simulink model "kinEq_sim_Explore_Badweh_2nd"  (R2024a)
settings: Solver=FixedStepDiscrete  StartTime=0.0  StopTime=5  FixedStep=TS  RelTol=1e-3  EnableMultiTasking=on
PostLoadFcn:
  | params
model workspace (MAT data in the model file):
  Ia = 0.1
  Id = 0.25
  Pa = 5
  Pd = 9
  TS = 0.01
undefined symbols (not defined in the file): DiscIntNeverNeededParam, L, r, sigbuilder_block, StartTheta, StartX, StartY
libraries: simulink_extras x9
settings Model: Creator=mgovinda  LastModifiedBy=Sheen
settings SolverCC: AlgebraicLoopSolver=TrustRegion
settings DataIOCC: LimitDataPoints=on  SaveFormat=Array  ReturnWorkspaceOutputs=off
settings OptimizationCC: LifeSpan=inf
settings DebuggingCC: UnconnectedInputMsg=warning  UnconnectedOutputMsg=warning  UnconnectedLineMsg=warning  SFUnexpectedBacktrackingDiag=warning  SFNoUnconditionalDefaultTransitionDiag=warning  SFExecutionAtInitializationDiag=none  ArithmeticOperatorsInVariantConditions=warning
settings HardwareCC: ProdBitPerPointer=32  ProdBitPerSizeT=32  ProdBitPerPtrDiffT=32  ProdLargestAtomicFloat=None  ProdIntDivRoundTo=Undefined  ProdEndianess=Unspecified  ProdWordSize=32  ProdHWDeviceType=32-bit Generic
settings ModelReferenceCC: EnableRefExpFcnMdlSchedulingChecks=on  PropagateSignalLabelsOutOfModel=off
settings SFSimCC: SimUseLocalCustomCode=off  CustomCodeUndefinedFunction=UseInterfaceOnly
settings RTWCC: RTWUseLocalCustomCode=off  GPUComputeCapability=3.5
settings CodeAppCC: StateflowObjectComments=on
settings GRTTargetCC: TargetLangStandard=C89/C90 (ANSI)
settings ConfigComp: CovMetricSettings=dw  CovSaveCumulativeToWorkspaceVar=on  CovSaveSingleToWorkspaceVar=on  CovExternalEMLEnable=off

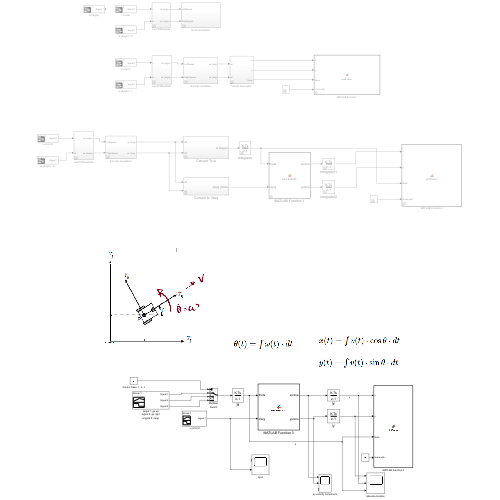
[thumbnail: Simulink's stored preview of the top-level diagram]
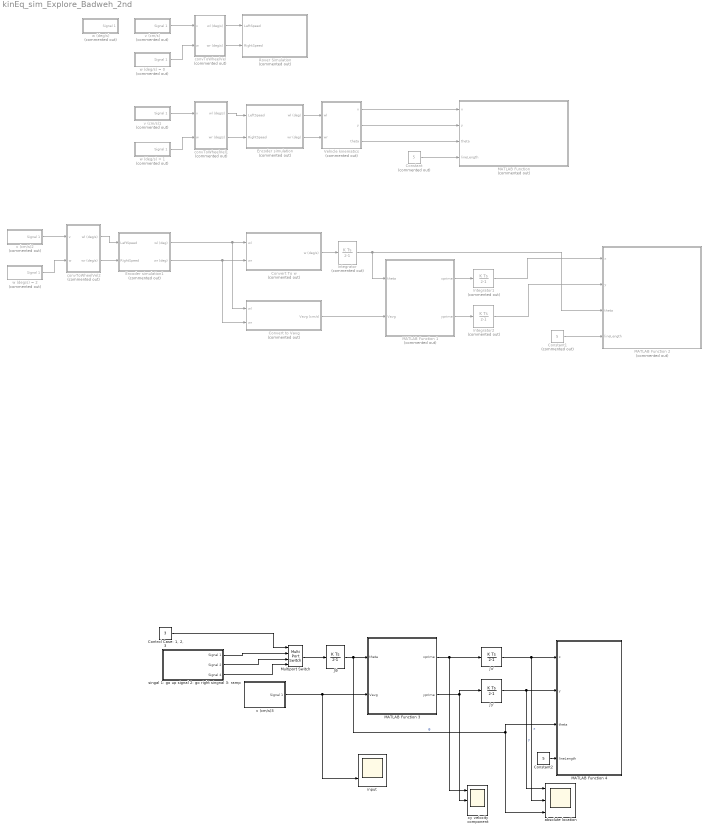
== system kinEq_sim_Explore_Badweh_2nd ==
  " Encoder simulation" : Subsystem  Commented=on
  " Encoder simulation1" : Subsystem  Commented=on
  Constant : Constant  Commented=on  Value=5
  Constant1 : Constant  Commented=on  Value=5
  Constant2 : Constant  Value=5
  "Control Case: 1, 2, 3" : Constant  Value=3
  Convert To w : Subsystem  Commented=on
  Convert to Vavg : Subsystem  Commented=on
  Integrator : DiscreteIntegrator  Commented=on  gainval=1  InitialCondition=StartTheta  SampleTime=-1  ICPrevOutput=DiscIntNeverNeededParam  ICPrevScaledInput=DiscIntNeverNeededParam
  Integrator1 : DiscreteIntegrator  Commented=on  gainval=1  InitialCondition=StartX  SampleTime=-1  ICPrevOutput=DiscIntNeverNeededParam  ICPrevScaledInput=DiscIntNeverNeededParam
  Integrator2 : DiscreteIntegrator  Commented=on  gainval=1  InitialCondition=StartY  SampleTime=-1  ICPrevOutput=DiscIntNeverNeededParam  ICPrevScaledInput=DiscIntNeverNeededParam
  "MATLAB Function " : MATLAB Function  Commented=on  TreatAsAtomicUnit=on
  MATLAB Function 1 : MATLAB Function  Commented=on  TreatAsAtomicUnit=on
  MATLAB Function 2 : MATLAB Function  Commented=on  TreatAsAtomicUnit=on
  MATLAB Function 3 : MATLAB Function  TreatAsAtomicUnit=on
  MATLAB Function 4 : MATLAB Function  TreatAsAtomicUnit=on
  "Multiport Switch " : MultiPortSwitch  SaturateOnIntegerOverflow=off  InputSameDT=off
  Rover Simulation : Subsystem  Commented=on
  Vehicle kinematics : Subsystem  Commented=on
  absolute location : Scope  NumInputPorts=3
  convToWheelVel : Subsystem  Commented=on
  convToWheelVel1 : Subsystem  Commented=on
  convToWheelVel2 : Subsystem  Commented=on
  input : Scope  NumInputPorts=2
  singal 1: go up signal 2: go right singnal 3: ramp : Subsystem  Tag=STV Subsys  LoadFcn=sigbuilder_block('load');  StartFcn=sigbuilder_block('start');  StopFcn=sigbuilder_block('stop');  ClipboardFcn=sigbuilder_block('clipboard');  mask(Sigbuilder block){tuvar=[0:10]}
      mask help: Simulink:masks:SigbuilderBlock_MD
      mask init:
      | if ~strcmp(get_param(bdroot(gcbh),'SimulationStatus'),'stopped') tuvar = sigbuilder_block('maskInit'); end
      settings: CopyFcn=sigbuilder_block('copy');  DeleteFcn=sigbuilder_block('delete');  ModelCloseFcn=sigbuilder_block('modelClose');  PreSaveFcn=sigbuilder_block('preSave');  PauseFcn=sigbuilder_block('pause');  ContinueFcn=sigbuilder_block('continue');  NameChangeFcn=sigbuilder_block('namechange');  OpenFcn=sigbuilder_block('open',[51 207.75 432.75 495.75 ]);  CloseFcn=sigbuilder_block('close');
      mask Display: plot(0, 0, 100, 100,[2, 2, 32, 32, 2], [68, 8, 8, 68, 68],[32, 2], [38, 38], [32, 19, 2],[53, 60, 44], [32, 17, 17, 2],[16, 16, 31, 31]);txt = getActiveGroup(gcbh);text(2, 100, txt,'verticalAlignment', 'top');
  v (cm/s) : Subsystem  Tag=STV Subsys  Commented=on  LoadFcn=sigbuilder_block('load');  StartFcn=sigbuilder_block('start');  StopFcn=sigbuilder_block('stop');  ClipboardFcn=sigbuilder_block('clipboard');  mask(Sigbuilder block){tuvar=[0:10]}
      mask help: Simulink:masks:SigbuilderBlock_MD
      mask init:
      | if ~strcmp(get_param(bdroot(gcbh),'SimulationStatus'),'stopped') tuvar = sigbuilder_block('maskInit'); end
      settings: CopyFcn=sigbuilder_block('copy');  DeleteFcn=sigbuilder_block('delete');  ModelCloseFcn=sigbuilder_block('modelClose');  PreSaveFcn=sigbuilder_block('preSave');  PauseFcn=sigbuilder_block('pause');  ContinueFcn=sigbuilder_block('continue');  NameChangeFcn=sigbuilder_block('namechange');  OpenFcn=sigbuilder_block('open',[2.25 144.75 600.75 275.25 ]);  CloseFcn=sigbuilder_block('close');
      mask Display: plot(0, 0, 100, 100,[2, 2, 32, 32, 2], [68, 8, 8, 68, 68],[32, 2], [38, 38], [32, 19, 2],[53, 60, 44], [32, 17, 17, 2],[16, 16, 31, 31]);txt = getActiveGroup(gcbh);text(2, 100, txt,'verticalAlignment', 'top');
  v (cm/s)1 : Subsystem  Tag=STV Subsys  Commented=on  LoadFcn=sigbuilder_block('load');  StartFcn=sigbuilder_block('start');  StopFcn=sigbuilder_block('stop');  ClipboardFcn=sigbuilder_block('clipboard');  mask(Sigbuilder block){tuvar=[0:10]}
      mask help: Simulink:masks:SigbuilderBlock_MD
      mask init:
      | if ~strcmp(get_param(bdroot(gcbh),'SimulationStatus'),'stopped') tuvar = sigbuilder_block('maskInit'); end
      settings: CopyFcn=sigbuilder_block('copy');  DeleteFcn=sigbuilder_block('delete');  ModelCloseFcn=sigbuilder_block('modelClose');  PreSaveFcn=sigbuilder_block('preSave');  PauseFcn=sigbuilder_block('pause');  ContinueFcn=sigbuilder_block('continue');  NameChangeFcn=sigbuilder_block('namechange');  OpenFcn=sigbuilder_block('open',[2.25 144.75 600.75 275.25 ]);  CloseFcn=sigbuilder_block('close');
      mask Display: plot(0, 0, 100, 100,[2, 2, 32, 32, 2], [68, 8, 8, 68, 68],[32, 2], [38, 38], [32, 19, 2],[53, 60, 44], [32, 17, 17, 2],[16, 16, 31, 31]);txt = getActiveGroup(gcbh);text(2, 100, txt,'verticalAlignment', 'top');
  v (cm/s)2 : Subsystem  Tag=STV Subsys  Commented=on  LoadFcn=sigbuilder_block('load');  StartFcn=sigbuilder_block('start');  StopFcn=sigbuilder_block('stop');  ClipboardFcn=sigbuilder_block('clipboard');  mask(Sigbuilder block){tuvar=[0:10]}
      mask help: Simulink:masks:SigbuilderBlock_MD
      mask init:
      | if ~strcmp(get_param(bdroot(gcbh),'SimulationStatus'),'stopped') tuvar = sigbuilder_block('maskInit'); end
      settings: CopyFcn=sigbuilder_block('copy');  DeleteFcn=sigbuilder_block('delete');  ModelCloseFcn=sigbuilder_block('modelClose');  PreSaveFcn=sigbuilder_block('preSave');  PauseFcn=sigbuilder_block('pause');  ContinueFcn=sigbuilder_block('continue');  NameChangeFcn=sigbuilder_block('namechange');  OpenFcn=sigbuilder_block('open',[2.25 144.75 600.75 275.25 ]);  CloseFcn=sigbuilder_block('close');
      mask Display: plot(0, 0, 100, 100,[2, 2, 32, 32, 2], [68, 8, 8, 68, 68],[32, 2], [38, 38], [32, 19, 2],[53, 60, 44], [32, 17, 17, 2],[16, 16, 31, 31]);txt = getActiveGroup(gcbh);text(2, 100, txt,'verticalAlignment', 'top');
  v (cm/s)3 : Subsystem  Tag=STV Subsys  LoadFcn=sigbuilder_block('load');  StartFcn=sigbuilder_block('start');  StopFcn=sigbuilder_block('stop');  ClipboardFcn=sigbuilder_block('clipboard');  mask(Sigbuilder block){tuvar=[0:10]}
      mask help: Simulink:masks:SigbuilderBlock_MD
      mask init:
      | if ~strcmp(get_param(bdroot(gcbh),'SimulationStatus'),'stopped') tuvar = sigbuilder_block('maskInit'); end
      settings: CopyFcn=sigbuilder_block('copy');  DeleteFcn=sigbuilder_block('delete');  ModelCloseFcn=sigbuilder_block('modelClose');  PreSaveFcn=sigbuilder_block('preSave');  PauseFcn=sigbuilder_block('pause');  ContinueFcn=sigbuilder_block('continue');  NameChangeFcn=sigbuilder_block('namechange');  OpenFcn=sigbuilder_block('open',[2.25 144.75 600.75 275.25 ]);  CloseFcn=sigbuilder_block('close');
      mask Display: plot(0, 0, 100, 100,[2, 2, 32, 32, 2], [68, 8, 8, 68, 68],[32, 2], [38, 38], [32, 19, 2],[53, 60, 44], [32, 17, 17, 2],[16, 16, 31, 31]);txt = getActiveGroup(gcbh);text(2, 100, txt,'verticalAlignment', 'top');
  w (deg/s) : Subsystem  Tag=STV Subsys  Commented=on  LoadFcn=sigbuilder_block('load');  StartFcn=sigbuilder_block('start');  StopFcn=sigbuilder_block('stop');  ClipboardFcn=sigbuilder_block('clipboard');  mask(Sigbuilder block){tuvar=[0:10]}
      mask help: Simulink:masks:SigbuilderBlock_MD
      mask init:
      | if ~strcmp(get_param(bdroot(gcbh),'SimulationStatus'),'stopped') tuvar = sigbuilder_block('maskInit'); end
      settings: CopyFcn=sigbuilder_block('copy');  DeleteFcn=sigbuilder_block('delete');  ModelCloseFcn=sigbuilder_block('modelClose');  PreSaveFcn=sigbuilder_block('preSave');  PauseFcn=sigbuilder_block('pause');  ContinueFcn=sigbuilder_block('continue');  NameChangeFcn=sigbuilder_block('namechange');  OpenFcn=sigbuilder_block('open',[210.75 142.5 475.5 277.5 ]);  CloseFcn=sigbuilder_block('close');
      mask Display: plot(0, 0, 100, 100,[2, 2, 32, 32, 2], [68, 8, 8, 68, 68],[32, 2], [38, 38], [32, 19, 2],[53, 60, 44], [32, 17, 17, 2],[16, 16, 31, 31]);txt = getActiveGroup(gcbh);text(2, 100, txt,'verticalAlignment', 'top');
  w (deg/s) = 0 : Subsystem  Tag=STV Subsys  Commented=on  LoadFcn=sigbuilder_block('load');  StartFcn=sigbuilder_block('start');  StopFcn=sigbuilder_block('stop');  ClipboardFcn=sigbuilder_block('clipboard');  mask(Sigbuilder block){tuvar=[0:10]}
      mask help: Simulink:masks:SigbuilderBlock_MD
      mask init:
      | if ~strcmp(get_param(bdroot(gcbh),'SimulationStatus'),'stopped') tuvar = sigbuilder_block('maskInit'); end
      settings: CopyFcn=sigbuilder_block('copy');  DeleteFcn=sigbuilder_block('delete');  ModelCloseFcn=sigbuilder_block('modelClose');  PreSaveFcn=sigbuilder_block('preSave');  PauseFcn=sigbuilder_block('pause');  ContinueFcn=sigbuilder_block('continue');  NameChangeFcn=sigbuilder_block('namechange');  OpenFcn=sigbuilder_block('open',[210.75 142.5 475.5 277.5 ]);  CloseFcn=sigbuilder_block('close');
      mask Display: plot(0, 0, 100, 100,[2, 2, 32, 32, 2], [68, 8, 8, 68, 68],[32, 2], [38, 38], [32, 19, 2],[53, 60, 44], [32, 17, 17, 2],[16, 16, 31, 31]);txt = getActiveGroup(gcbh);text(2, 100, txt,'verticalAlignment', 'top');
  w (deg/s) = 1 : Subsystem  Tag=STV Subsys  Commented=on  LoadFcn=sigbuilder_block('load');  StartFcn=sigbuilder_block('start');  StopFcn=sigbuilder_block('stop');  ClipboardFcn=sigbuilder_block('clipboard');  mask(Sigbuilder block){tuvar=[0:10]}
      mask help: Simulink:masks:SigbuilderBlock_MD
      mask init:
      | if ~strcmp(get_param(bdroot(gcbh),'SimulationStatus'),'stopped') tuvar = sigbuilder_block('maskInit'); end
      settings: CopyFcn=sigbuilder_block('copy');  DeleteFcn=sigbuilder_block('delete');  ModelCloseFcn=sigbuilder_block('modelClose');  PreSaveFcn=sigbuilder_block('preSave');  PauseFcn=sigbuilder_block('pause');  ContinueFcn=sigbuilder_block('continue');  NameChangeFcn=sigbuilder_block('namechange');  OpenFcn=sigbuilder_block('open',[210.75 142.5 475.5 277.5 ]);  CloseFcn=sigbuilder_block('close');
      mask Display: plot(0, 0, 100, 100,[2, 2, 32, 32, 2], [68, 8, 8, 68, 68],[32, 2], [38, 38], [32, 19, 2],[53, 60, 44], [32, 17, 17, 2],[16, 16, 31, 31]);txt = getActiveGroup(gcbh);text(2, 100, txt,'verticalAlignment', 'top');
  w (deg/s) = 2 : Subsystem  Tag=STV Subsys  Commented=on  LoadFcn=sigbuilder_block('load');  StartFcn=sigbuilder_block('start');  StopFcn=sigbuilder_block('stop');  ClipboardFcn=sigbuilder_block('clipboard');  mask(Sigbuilder block){tuvar=[0:10]}
      mask help: Simulink:masks:SigbuilderBlock_MD
      mask init:
      | if ~strcmp(get_param(bdroot(gcbh),'SimulationStatus'),'stopped') tuvar = sigbuilder_block('maskInit'); end
      settings: CopyFcn=sigbuilder_block('copy');  DeleteFcn=sigbuilder_block('delete');  ModelCloseFcn=sigbuilder_block('modelClose');  PreSaveFcn=sigbuilder_block('preSave');  PauseFcn=sigbuilder_block('pause');  ContinueFcn=sigbuilder_block('continue');  NameChangeFcn=sigbuilder_block('namechange');  OpenFcn=sigbuilder_block('open',[210.75 142.5 475.5 277.5 ]);  CloseFcn=sigbuilder_block('close');
      mask Display: plot(0, 0, 100, 100,[2, 2, 32, 32, 2], [68, 8, 8, 68, 68],[32, 2], [38, 38], [32, 19, 2],[53, 60, 44], [32, 17, 17, 2],[16, 16, 31, 31]);txt = getActiveGroup(gcbh);text(2, 100, txt,'verticalAlignment', 'top');
  xy velocity component : Scope  NumInputPorts=3
  ∫x' : DiscreteIntegrator  gainval=1  InitialCondition=StartX  SampleTime=-1  ICPrevOutput=DiscIntNeverNeededParam  ICPrevScaledInput=DiscIntNeverNeededParam
  ∫y' : DiscreteIntegrator  gainval=1  InitialCondition=StartY  SampleTime=-1  ICPrevOutput=DiscIntNeverNeededParam  ICPrevScaledInput=DiscIntNeverNeededParam
  ∫θ : DiscreteIntegrator  gainval=1  InitialCondition=StartTheta  SampleTime=-1  ICPrevOutput=DiscIntNeverNeededParam  ICPrevScaledInput=DiscIntNeverNeededParam
  wires:
  convToWheelVel/1(wl (deg/s)) -> Rover Simulation/1(LeftSpeed)
  convToWheelVel/2(wr (deg/s)) -> Rover Simulation/2(RightSpeed)
  v (cm/s)/1(Signal 1) -> convToWheelVel/1(v)
  w (deg/s) = 0/1(Signal 1) -> convToWheelVel/2(w)
  w (deg/s) = 1/1(Signal 1) -> convToWheelVel1/2(w)
  v (cm/s)1/1(Signal 1) -> convToWheelVel1/1(v)
  " Encoder simulation"/2(wr (deg)) -> Vehicle kinematics/2(wr)
  " Encoder simulation"/1(wl (deg)) -> Vehicle kinematics/1(wl)
  convToWheelVel1/1(wl (deg/s)) -> " Encoder simulation"/1(LeftSpeed)
  convToWheelVel1/2(wr (deg/s)) -> " Encoder simulation"/2(RightSpeed)
  Constant/1 -> "MATLAB Function "/4(lineLength)
  Vehicle kinematics/2(y) -> "MATLAB Function "/2(y)
  Vehicle kinematics/1(x) -> "MATLAB Function "/1(x)
  Vehicle kinematics/3(theta) -> "MATLAB Function "/3(theta)
  MATLAB Function 1/1(xprime) -> Integrator1/1
  Integrator/1 -> MATLAB Function 2/3(theta), MATLAB Function 1/1(theta)
  Integrator2/1 -> MATLAB Function 2/2(y)
  Convert to Vavg/1(Vavg (cm/s)) -> MATLAB Function 1/2(Vavg)
  " Encoder simulation1"/1(wl (deg)) -> Convert to Vavg/1(wl), Convert To w/1(wl)
  " Encoder simulation1"/2(wr (deg)) -> Convert to Vavg/2(wr), Convert To w/2(wr)
  Convert To w/1(w (deg/s)) -> Integrator/1
  Integrator1/1 -> MATLAB Function 2/1(x)
  MATLAB Function 1/2(yprime) -> Integrator2/1
  v (cm/s)2/1(Signal 1) -> convToWheelVel2/1(v)
  w (deg/s) = 2/1(Signal 1) -> convToWheelVel2/2(w)
  convToWheelVel2/1(wl (deg/s)) -> " Encoder simulation1"/1(LeftSpeed)
  convToWheelVel2/2(wr (deg/s)) -> " Encoder simulation1"/2(RightSpeed)
  Constant1/1 -> MATLAB Function 2/4(lineLength)
  ∫y'/1 -> absolute location/1, MATLAB Function 4/2(y)  "y"
  ∫x'/1 -> MATLAB Function 4/1(x), absolute location/2  "x"
  MATLAB Function 3/2(yprime) -> xy velocity component/2, ∫y'/1
  ∫θ/1 -> absolute location/3, MATLAB Function 4/3(theta), MATLAB Function 3/1(theta)  "θ"
  Constant2/1 -> MATLAB Function 4/4(lineLength)
  MATLAB Function 3/1(xprime) -> xy velocity component/1, ∫x'/1
  v (cm/s)3/1(Signal 1) -> input/2, MATLAB Function 3/2(Vavg)
  "Multiport Switch "/1 -> ∫θ/1
  singal 1: go up signal 2: go right singnal 3: ramp/1(Signal 1) -> "Multiport Switch "/2
  singal 1: go up signal 2: go right singnal 3: ramp/2(Signal 2) -> "Multiport Switch "/3
  "Control Case: 1, 2, 3"/1 -> "Multiport Switch "/1
  singal 1: go up signal 2: go right singnal 3: ramp/3(Signal 4) -> "Multiport Switch "/4

== system kinEq_sim_Explore_Badweh_2nd/ Encoder simulation ==
  note: Assumption - The desired speed is the actual speed of the wheels
  LeftSpeed : Inport
  RightSpeed : Inport  Port=2
  Encoder : Subsystem
  wl (deg) : Outport  VectorParamsAs1DForOutWhenUnconnected=off
  wr (deg) : Outport  Port=2  VectorParamsAs1DForOutWhenUnconnected=off
  wires:
  Encoder/1(LDegrees) -> wl (deg)/1
  Encoder/2(RDegrees) -> wr (deg)/1
  RightSpeed/1 -> Encoder/2(Rwheelspeed)
  LeftSpeed/1 -> Encoder/1(Lwheelspeed)

== system kinEq_sim_Explore_Badweh_2nd/ Encoder simulation1 ==
  note: Assumption - The desired speed is the actual speed of the wheels
  LeftSpeed : Inport
  RightSpeed : Inport  Port=2
  Encoder : Subsystem
  wl (deg) : Outport  VectorParamsAs1DForOutWhenUnconnected=off
  wr (deg) : Outport  Port=2  VectorParamsAs1DForOutWhenUnconnected=off
  wires:
  Encoder/1(LDegrees) -> wl (deg)/1
  Encoder/2(RDegrees) -> wr (deg)/1
  RightSpeed/1 -> Encoder/2(Rwheelspeed)
  LeftSpeed/1 -> Encoder/1(Lwheelspeed)

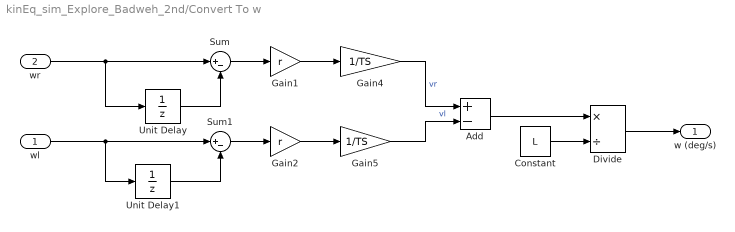
== system kinEq_sim_Explore_Badweh_2nd/Convert To w ==
  wl : Inport
  wr : Inport  Port=2
  Add : Sum  Inputs=+-
  Constant : Constant  Value=L
  Divide : Product  Inputs=*/
  Gain1 : Gain  Gain=r
  Gain2 : Gain  Gain=r
  Gain4 : Gain  Gain=1/TS
  Gain5 : Gain  Gain=1/TS
  Sum : Sum  Inputs=|+-
  Sum1 : Sum  Inputs=|+-
  Unit Delay : UnitDelay  SampleTime=-1  HasFrameUpgradeWarning=on
  Unit Delay1 : UnitDelay  SampleTime=-1  HasFrameUpgradeWarning=on
  w (deg/s) : Outport  VectorParamsAs1DForOutWhenUnconnected=off
  wires:
  Unit Delay1/1 -> Sum1/2
  Sum1/1 -> Gain2/1
  wl/1 -> Sum1/1, Unit Delay1/1
  wr/1 -> Sum/1, Unit Delay/1
  Sum/1 -> Gain1/1
  Unit Delay/1 -> Sum/2
  Gain1/1 -> Gain4/1
  Gain2/1 -> Gain5/1
  Add/1 -> Divide/1
  Constant/1 -> Divide/2
  Gain4/1 -> Add/1  "vr"
  Gain5/1 -> Add/2  "vl"
  Divide/1 -> w (deg/s)/1

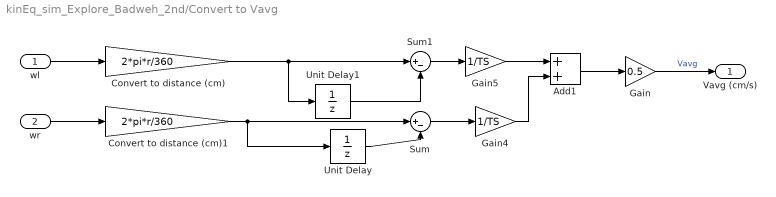
== system kinEq_sim_Explore_Badweh_2nd/Convert to Vavg ==
  wl : Inport
  wr : Inport  Port=2
  Add1 : Sum
  Convert to distance (cm) : Gain  Gain=2*pi*r/360
  Convert to distance (cm)1 : Gain  Gain=2*pi*r/360
  Gain : Gain  Gain=0.5
  Gain4 : Gain  Gain=1/TS
  Gain5 : Gain  Gain=1/TS
  Sum : Sum  Inputs=|+-
  Sum1 : Sum  Inputs=|+-
  Unit Delay : UnitDelay  SampleTime=-1  HasFrameUpgradeWarning=on
  Unit Delay1 : UnitDelay  SampleTime=-1  HasFrameUpgradeWarning=on
  Vavg (cm/s) : Outport  VectorParamsAs1DForOutWhenUnconnected=off
  wires:
  Gain/1 -> Vavg (cm/s)/1  "Vavg"
  Add1/1 -> Gain/1
  Unit Delay/1 -> Sum/2
  Sum/1 -> Gain4/1
  wr/1 -> Convert to distance (cm)1/1
  Gain4/1 -> Add1/2
  Gain5/1 -> Add1/1
  Sum1/1 -> Gain5/1
  Unit Delay1/1 -> Sum1/2
  wl/1 -> Convert to distance (cm)/1
  Convert to distance (cm)/1 -> Unit Delay1/1, Sum1/1
  Convert to distance (cm)1/1 -> Unit Delay/1, Sum/1

== system kinEq_sim_Explore_Badweh_2nd/Rover Simulation ==
  LeftSpeed : Inport
  RightSpeed : Inport  Port=2
  " Encoder simulation" : Subsystem
  Robot path plotter : Subsystem
  Vehicle kinematics : Subsystem
  wires:
  Vehicle kinematics/1(x) -> Robot path plotter/1(X)
  Vehicle kinematics/2(y) -> Robot path plotter/2(Y)
  Vehicle kinematics/3(theta) -> Robot path plotter/3(theta)
  LeftSpeed/1 -> " Encoder simulation"/1(LeftSpeed)
  RightSpeed/1 -> " Encoder simulation"/2(RightSpeed)
  " Encoder simulation"/1(wl (deg)) -> Vehicle kinematics/1(wl)
  " Encoder simulation"/2(wr (deg)) -> Vehicle kinematics/2(wr)

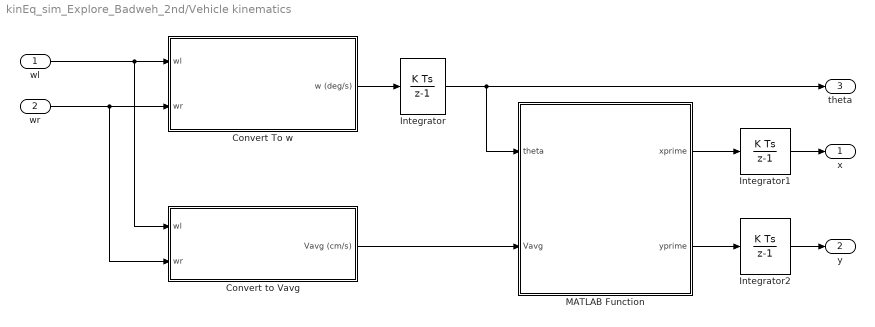
== system kinEq_sim_Explore_Badweh_2nd/Vehicle kinematics ==
  wl : Inport
  wr : Inport  Port=2
  Convert To w : Subsystem
  Convert to Vavg : Subsystem
  Integrator : DiscreteIntegrator  gainval=1  InitialCondition=StartTheta  SampleTime=-1  ICPrevOutput=DiscIntNeverNeededParam  ICPrevScaledInput=DiscIntNeverNeededParam
  Integrator1 : DiscreteIntegrator  gainval=1  InitialCondition=StartX  SampleTime=-1  ICPrevOutput=DiscIntNeverNeededParam  ICPrevScaledInput=DiscIntNeverNeededParam
  Integrator2 : DiscreteIntegrator  gainval=1  InitialCondition=StartY  SampleTime=-1  ICPrevOutput=DiscIntNeverNeededParam  ICPrevScaledInput=DiscIntNeverNeededParam
  "MATLAB Function " : MATLAB Function  TreatAsAtomicUnit=on
  x : Outport  VectorParamsAs1DForOutWhenUnconnected=off
  y : Outport  Port=2  VectorParamsAs1DForOutWhenUnconnected=off
  theta : Outport  Port=3  VectorParamsAs1DForOutWhenUnconnected=off
  wires:
  "MATLAB Function "/1(xprime) -> Integrator1/1
  "MATLAB Function "/2(yprime) -> Integrator2/1
  Integrator1/1 -> x/1
  Integrator2/1 -> y/1
  Integrator/1 -> theta/1, "MATLAB Function "/1(theta)
  wl/1 -> Convert to Vavg/1(wl), Convert To w/1(wl)
  wr/1 -> Convert to Vavg/2(wr), Convert To w/2(wr)
  Convert to Vavg/1(Vavg (cm/s)) -> "MATLAB Function "/2(Vavg)
  Convert To w/1(w (deg/s)) -> Integrator/1

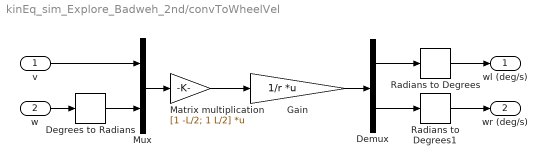
== system kinEq_sim_Explore_Badweh_2nd/convToWheelVel ==
  v : Inport
  w : Inport  Port=2
  " Gain" : Gain  Gain=1/r  Multiplication=Matrix(K*u)
  Degrees to Radians : simulink_extras/Transformations/Degrees to Radians
  Demux : Demux  Outputs=2
  Matrix multiplication : Gain  Gain=[1 -L/2; 1 L/2]  Multiplication=Matrix(K*u)
  Mux : Mux  Inputs=2
  Radians to Degrees : simulink_extras/Transformations/Radians to Degrees
  Radians to Degrees1 : simulink_extras/Transformations/Radians to Degrees
  wl (deg/s) : Outport  VectorParamsAs1DForOutWhenUnconnected=off
  wr (deg/s) : Outport  Port=2  VectorParamsAs1DForOutWhenUnconnected=off
  wires:
  " Gain"/1 -> Demux/1
  Matrix multiplication/1 -> " Gain"/1
  v/1 -> Mux/1
  Mux/1 -> Matrix multiplication/1
  Demux/1 -> Radians to Degrees/1
  Demux/2 -> Radians to Degrees1/1
  w/1 -> Degrees to Radians/1
  Radians to Degrees/1 -> wl (deg/s)/1
  Radians to Degrees1/1 -> wr (deg/s)/1
  Degrees to Radians/1 -> Mux/2

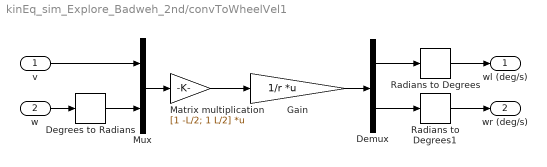
== system kinEq_sim_Explore_Badweh_2nd/convToWheelVel1 ==
  v : Inport
  w : Inport  Port=2
  " Gain" : Gain  Gain=1/r  Multiplication=Matrix(K*u)
  Degrees to Radians : simulink_extras/Transformations/Degrees to Radians
  Demux : Demux  Outputs=2
  Matrix multiplication : Gain  Gain=[1 -L/2; 1 L/2]  Multiplication=Matrix(K*u)
  Mux : Mux  Inputs=2
  Radians to Degrees : simulink_extras/Transformations/Radians to Degrees
  Radians to Degrees1 : simulink_extras/Transformations/Radians to Degrees
  wl (deg/s) : Outport  VectorParamsAs1DForOutWhenUnconnected=off
  wr (deg/s) : Outport  Port=2  VectorParamsAs1DForOutWhenUnconnected=off
  wires:
  " Gain"/1 -> Demux/1
  Matrix multiplication/1 -> " Gain"/1
  v/1 -> Mux/1
  Mux/1 -> Matrix multiplication/1
  Demux/1 -> Radians to Degrees/1
  Demux/2 -> Radians to Degrees1/1
  w/1 -> Degrees to Radians/1
  Radians to Degrees/1 -> wl (deg/s)/1
  Radians to Degrees1/1 -> wr (deg/s)/1
  Degrees to Radians/1 -> Mux/2

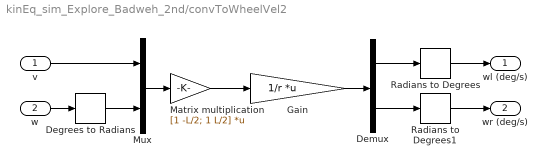
== system kinEq_sim_Explore_Badweh_2nd/convToWheelVel2 ==
  v : Inport
  w : Inport  Port=2
  " Gain" : Gain  Gain=1/r  Multiplication=Matrix(K*u)
  Degrees to Radians : simulink_extras/Transformations/Degrees to Radians
  Demux : Demux  Outputs=2
  Matrix multiplication : Gain  Gain=[1 -L/2; 1 L/2]  Multiplication=Matrix(K*u)
  Mux : Mux  Inputs=2
  Radians to Degrees : simulink_extras/Transformations/Radians to Degrees
  Radians to Degrees1 : simulink_extras/Transformations/Radians to Degrees
  wl (deg/s) : Outport  VectorParamsAs1DForOutWhenUnconnected=off
  wr (deg/s) : Outport  Port=2  VectorParamsAs1DForOutWhenUnconnected=off
  wires:
  " Gain"/1 -> Demux/1
  Matrix multiplication/1 -> " Gain"/1
  v/1 -> Mux/1
  Mux/1 -> Matrix multiplication/1
  Demux/1 -> Radians to Degrees/1
  Demux/2 -> Radians to Degrees1/1
  w/1 -> Degrees to Radians/1
  Radians to Degrees/1 -> wl (deg/s)/1
  Radians to Degrees1/1 -> wr (deg/s)/1
  Degrees to Radians/1 -> Mux/2

== system kinEq_sim_Explore_Badweh_2nd/singal 1: go up signal 2: go right singnal 3: ramp ==
  Demux : Demux  Tag=STV Demux  Outputs=3
      settings: DisplayOption=none
  FromWs : FromWorkspace  Tag=STV FromWs  VariableName=tuvar
      SigBuilderData=|
      | common.afterFinalStr = 'Extrapolate'
      | common.sampleTime = 0
      | dataSet.timeRange = [0 11]
      | dataSet.name = 'Group 1'
      | sbobj.Groups.Name = 'Group 1'
      | sbobj.Groups.Signals(1).Name = 'Signal 1'
      | sbobj.Groups.Signals(1).XData = [0 5 10 11]
      | sbobj.Groups.Signals(1).YData = [0 0 0 0]
      | sbobj.Groups.Signals(2).Name = 'Signal 2'
      | sbobj.Groups.Signals(2).XData = [0 1.02 1.02 11]
      | sbobj.Groups.Signals(2).YData = [-90 -90 0 0]
      | sbobj.Groups.Signals(3).Name = 'Signal 4'
      | sbobj.Groups.Signals(3).XData = [0 1 1 11]
      | sbobj.Groups.Signals(3).YData = [-45 -45 0 0]
      | sbobj.Groups.TimeRange = [0 11]
  Signal 1 : Outport  Tag=STV Outport  VectorParamsAs1DForOutWhenUnconnected=off
  Signal 2 : Outport  Tag=STV Outport  Port=2
  Signal 4 : Outport  Tag=STV Outport  Port=3
  wires:
  Demux/1 -> Signal 1/1
  FromWs/1 -> Demux/1
  Demux/2 -> Signal 2/1
  Demux/3 -> Signal 4/1

== system kinEq_sim_Explore_Badweh_2nd/v (cm//s) ==
  Demux : Demux  Tag=STV Demux  Outputs=1
      settings: DisplayOption=none
  FromWs : FromWorkspace  Tag=STV FromWs  VariableName=tuvar
      SigBuilderData=|
      | common.afterFinalStr = 'Extrapolate'
      | common.sampleTime = 0
      | dataSet.timeRange = [0 10]
      | dataSet.name = 'Group 1'
      | sbobj.Groups.Name = 'Group 1'
      | sbobj.Groups.Signals.Name = 'Signal 1'
      | sbobj.Groups.Signals.XData = [0 5 5 6 10]
      | sbobj.Groups.Signals.YData = [10 10 0 0 0]
  Signal 1 : Outport  Tag=STV Outport  VectorParamsAs1DForOutWhenUnconnected=off
  wires:
  Demux/1 -> Signal 1/1
  FromWs/1 -> Demux/1

== system kinEq_sim_Explore_Badweh_2nd/v (cm//s)1 ==
  Demux : Demux  Tag=STV Demux  Outputs=1
      settings: DisplayOption=none
  FromWs : FromWorkspace  Tag=STV FromWs  VariableName=tuvar
      SigBuilderData=|
      | common.afterFinalStr = 'Extrapolate'
      | common.sampleTime = 0
      | dataSet.timeRange = [0 10]
      | dataSet.name = 'Group 1'
      | sbobj.Groups.Name = 'Group 1'
      | sbobj.Groups.Signals.Name = 'Signal 1'
      | sbobj.Groups.Signals.XData = [0 5 5 6 10]
      | sbobj.Groups.Signals.YData = [10 10 0 0 0]
  Signal 1 : Outport  Tag=STV Outport  VectorParamsAs1DForOutWhenUnconnected=off
  wires:
  Demux/1 -> Signal 1/1
  FromWs/1 -> Demux/1

== system kinEq_sim_Explore_Badweh_2nd/v (cm//s)2 ==
  Demux : Demux  Tag=STV Demux  Outputs=1
      settings: DisplayOption=none
  FromWs : FromWorkspace  Tag=STV FromWs  VariableName=tuvar
      SigBuilderData=|
      | common.afterFinalStr = 'Extrapolate'
      | common.sampleTime = 0
      | dataSet.timeRange = [0 10]
      | dataSet.name = 'Group 1'
      | sbobj.Groups.Name = 'Group 1'
      | sbobj.Groups.Signals.Name = 'Signal 1'
      | sbobj.Groups.Signals.XData = [0 5 5 6 10]
      | sbobj.Groups.Signals.YData = [10 10 0 0 0]
  Signal 1 : Outport  Tag=STV Outport  VectorParamsAs1DForOutWhenUnconnected=off
  wires:
  Demux/1 -> Signal 1/1
  FromWs/1 -> Demux/1

== system kinEq_sim_Explore_Badweh_2nd/v (cm//s)3 ==
  Demux : Demux  Tag=STV Demux  Outputs=1
      settings: DisplayOption=none
  FromWs : FromWorkspace  Tag=STV FromWs  VariableName=tuvar
      SigBuilderData=|
      | common.afterFinalStr = 'Extrapolate'
      | common.sampleTime = 0
      | dataSet.timeRange = [0 10]
      | dataSet.name = 'Group 1'
      | sbobj.Groups.Name = 'Group 1'
      | sbobj.Groups.Signals.Name = 'Signal 1'
      | sbobj.Groups.Signals.XData = [0 5 5 6 10]
      | sbobj.Groups.Signals.YData = [10 10 0 0 0]
  Signal 1 : Outport  Tag=STV Outport  VectorParamsAs1DForOutWhenUnconnected=off
  wires:
  Demux/1 -> Signal 1/1
  FromWs/1 -> Demux/1

== system kinEq_sim_Explore_Badweh_2nd/w (deg//s) ==
  Demux : Demux  Tag=STV Demux  Outputs=1
      settings: DisplayOption=none
  FromWs : FromWorkspace  Tag=STV FromWs  VariableName=tuvar
      SigBuilderData=|
      | common.afterFinalStr = 'Extrapolate'
      | common.sampleTime = 0
      | dataSet.timeRange = [0 11]
      | dataSet.name = 'Group 1'
      | sbobj.Groups.Name = 'Group 1'
      | sbobj.Groups.Signals.Name = 'Signal 1'
      | sbobj.Groups.Signals.XData = [0 5 5 10 10 11]
      | sbobj.Groups.Signals.YData = [0 0 72 72 0 0]
      | sbobj.Groups.TimeRange = [0 11]
  Signal 1 : Outport  Tag=STV Outport  VectorParamsAs1DForOutWhenUnconnected=off
  wires:
  FromWs/1 -> Demux/1
  Demux/1 -> Signal 1/1

== system kinEq_sim_Explore_Badweh_2nd/w (deg//s) = 0 ==
  Demux : Demux  Tag=STV Demux  Outputs=1
      settings: DisplayOption=none
  FromWs : FromWorkspace  Tag=STV FromWs  VariableName=tuvar
      SigBuilderData=|
      | common.afterFinalStr = 'Extrapolate'
      | common.sampleTime = 0
      | dataSet.timeRange = [0 11]
      | dataSet.name = 'Group 1'
      | sbobj.Groups.Name = 'Group 1'
      | sbobj.Groups.Signals.Name = 'Signal 1'
      | sbobj.Groups.Signals.XData = [0 5 5 10 10 11]
      | sbobj.Groups.Signals.YData = [0 0 0 0 0 0]
      | sbobj.Groups.TimeRange = [0 11]
  Signal 1 : Outport  Tag=STV Outport  VectorParamsAs1DForOutWhenUnconnected=off
  wires:
  Demux/1 -> Signal 1/1
  FromWs/1 -> Demux/1

== system kinEq_sim_Explore_Badweh_2nd/w (deg//s) = 1 ==
  Demux : Demux  Tag=STV Demux  Outputs=1
      settings: DisplayOption=none
  FromWs : FromWorkspace  Tag=STV FromWs  VariableName=tuvar
      SigBuilderData=|
      | common.afterFinalStr = 'Extrapolate'
      | common.sampleTime = 0
      | dataSet.timeRange = [0 11]
      | dataSet.name = 'Group 1'
      | sbobj.Groups.Name = 'Group 1'
      | sbobj.Groups.Signals.Name = 'Signal 1'
      | sbobj.Groups.Signals.XData = [0 5 5 10 10 11]
      | sbobj.Groups.Signals.YData = [0 0 0 0 0 0]
      | sbobj.Groups.TimeRange = [0 11]
  Signal 1 : Outport  Tag=STV Outport  VectorParamsAs1DForOutWhenUnconnected=off
  wires:
  Demux/1 -> Signal 1/1
  FromWs/1 -> Demux/1

== system kinEq_sim_Explore_Badweh_2nd/w (deg//s) = 2 ==
  Demux : Demux  Tag=STV Demux  Outputs=1
      settings: DisplayOption=none
  FromWs : FromWorkspace  Tag=STV FromWs  VariableName=tuvar
      SigBuilderData=|
      | common.afterFinalStr = 'Extrapolate'
      | common.sampleTime = 0
      | dataSet.timeRange = [0 11]
      | dataSet.name = 'Group 1'
      | sbobj.Groups.Name = 'Group 1'
      | sbobj.Groups.Signals.Name = 'Signal 1'
      | sbobj.Groups.Signals.XData = [0 5 5 10 10 11]
      | sbobj.Groups.Signals.YData = [0 0 0 0 0 0]
      | sbobj.Groups.TimeRange = [0 11]
  Signal 1 : Outport  Tag=STV Outport  VectorParamsAs1DForOutWhenUnconnected=off
  wires:
  Demux/1 -> Signal 1/1
  FromWs/1 -> Demux/1

== system kinEq_sim_Explore_Badweh_2nd/ Encoder simulation/Encoder ==
  Lwheelspeed : Inport
  Rwheelspeed : Inport  Port=2
  Discrete-Time Integrator : DiscreteIntegrator  SampleTime=-1  ICPrevOutput=DiscIntNeverNeededParam  ICPrevScaledInput=DiscIntNeverNeededParam
  Discrete-Time Integrator1 : DiscreteIntegrator  SampleTime=-1  ICPrevOutput=DiscIntNeverNeededParam  ICPrevScaledInput=DiscIntNeverNeededParam
  LDegrees : Outport  VectorParamsAs1DForOutWhenUnconnected=off
  RDegrees : Outport  Port=2  VectorParamsAs1DForOutWhenUnconnected=off
  wires:
  Rwheelspeed/1 -> Discrete-Time Integrator/1
  Lwheelspeed/1 -> Discrete-Time Integrator1/1
  Discrete-Time Integrator/1 -> RDegrees/1
  Discrete-Time Integrator1/1 -> LDegrees/1

== system kinEq_sim_Explore_Badweh_2nd/ Encoder simulation1/Encoder ==
  Lwheelspeed : Inport
  Rwheelspeed : Inport  Port=2
  Discrete-Time Integrator : DiscreteIntegrator  SampleTime=-1  ICPrevOutput=DiscIntNeverNeededParam  ICPrevScaledInput=DiscIntNeverNeededParam
  Discrete-Time Integrator1 : DiscreteIntegrator  SampleTime=-1  ICPrevOutput=DiscIntNeverNeededParam  ICPrevScaledInput=DiscIntNeverNeededParam
  LDegrees : Outport  VectorParamsAs1DForOutWhenUnconnected=off
  RDegrees : Outport  Port=2  VectorParamsAs1DForOutWhenUnconnected=off
  wires:
  Rwheelspeed/1 -> Discrete-Time Integrator/1
  Lwheelspeed/1 -> Discrete-Time Integrator1/1
  Discrete-Time Integrator/1 -> RDegrees/1
  Discrete-Time Integrator1/1 -> LDegrees/1

== system kinEq_sim_Explore_Badweh_2nd/Rover Simulation/ Encoder simulation ==
  note: Assumption - The desired speed is the actual speed of the wheels
  LeftSpeed : Inport
  RightSpeed : Inport  Port=2
  Encoder : Subsystem
  wl (deg) : Outport  VectorParamsAs1DForOutWhenUnconnected=off
  wr (deg) : Outport  Port=2  VectorParamsAs1DForOutWhenUnconnected=off
  wires:
  Encoder/1(LDegrees) -> wl (deg)/1
  Encoder/2(RDegrees) -> wr (deg)/1
  RightSpeed/1 -> Encoder/2(Rwheelspeed)
  LeftSpeed/1 -> Encoder/1(Lwheelspeed)

== system kinEq_sim_Explore_Badweh_2nd/Rover Simulation/Robot path plotter ==
  X : Inport
  Y : Inport  Port=2
  theta : Inport  Port=3
  Constant : Constant  Value=5
  "MATLAB Function " : MATLAB Function  TreatAsAtomicUnit=on
  wires:
  Constant/1 -> "MATLAB Function "/4(lineLength)
  X/1 -> "MATLAB Function "/1(x)
  Y/1 -> "MATLAB Function "/2(y)
  theta/1 -> "MATLAB Function "/3(theta)

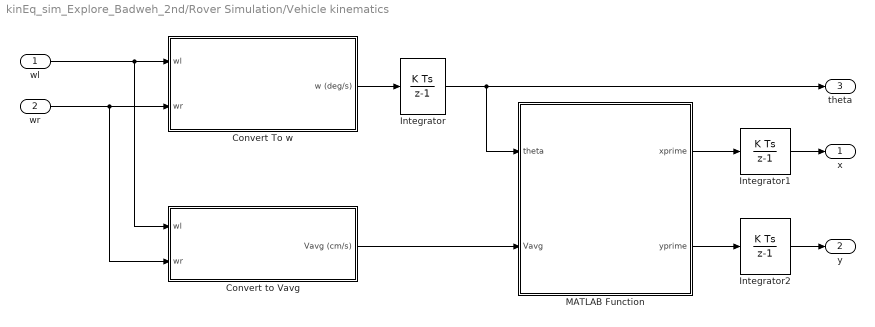
== system kinEq_sim_Explore_Badweh_2nd/Rover Simulation/Vehicle kinematics ==
  wl : Inport
  wr : Inport  Port=2
  Convert To w : Subsystem
  Convert to Vavg : Subsystem
  Integrator : DiscreteIntegrator  gainval=1  InitialCondition=StartTheta  SampleTime=-1  ICPrevOutput=DiscIntNeverNeededParam  ICPrevScaledInput=DiscIntNeverNeededParam
  Integrator1 : DiscreteIntegrator  gainval=1  InitialCondition=StartX  SampleTime=-1  ICPrevOutput=DiscIntNeverNeededParam  ICPrevScaledInput=DiscIntNeverNeededParam
  Integrator2 : DiscreteIntegrator  gainval=1  InitialCondition=StartY  SampleTime=-1  ICPrevOutput=DiscIntNeverNeededParam  ICPrevScaledInput=DiscIntNeverNeededParam
  "MATLAB Function " : MATLAB Function  TreatAsAtomicUnit=on
  x : Outport  VectorParamsAs1DForOutWhenUnconnected=off
  y : Outport  Port=2  VectorParamsAs1DForOutWhenUnconnected=off
  theta : Outport  Port=3  VectorParamsAs1DForOutWhenUnconnected=off
  wires:
  "MATLAB Function "/1(xprime) -> Integrator1/1
  "MATLAB Function "/2(yprime) -> Integrator2/1
  Integrator1/1 -> x/1
  Integrator2/1 -> y/1
  Integrator/1 -> theta/1, "MATLAB Function "/1(theta)
  wl/1 -> Convert to Vavg/1(wl), Convert To w/1(wl)
  wr/1 -> Convert to Vavg/2(wr), Convert To w/2(wr)
  Convert to Vavg/1(Vavg (cm/s)) -> "MATLAB Function "/2(Vavg)
  Convert To w/1(w (deg/s)) -> Integrator/1

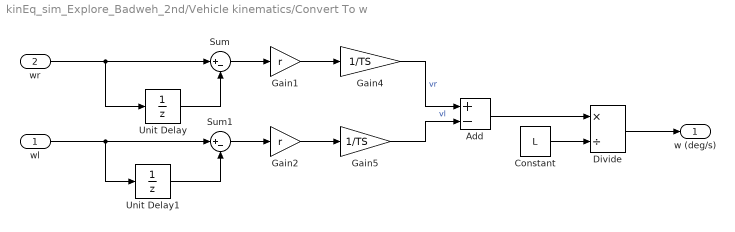
== system kinEq_sim_Explore_Badweh_2nd/Vehicle kinematics/Convert To w ==
  wl : Inport
  wr : Inport  Port=2
  Add : Sum  Inputs=+-
  Constant : Constant  Value=L
  Divide : Product  Inputs=*/
  Gain1 : Gain  Gain=r
  Gain2 : Gain  Gain=r
  Gain4 : Gain  Gain=1/TS
  Gain5 : Gain  Gain=1/TS
  Sum : Sum  Inputs=|+-
  Sum1 : Sum  Inputs=|+-
  Unit Delay : UnitDelay  SampleTime=-1  HasFrameUpgradeWarning=on
  Unit Delay1 : UnitDelay  SampleTime=-1  HasFrameUpgradeWarning=on
  w (deg/s) : Outport  VectorParamsAs1DForOutWhenUnconnected=off
  wires:
  Unit Delay1/1 -> Sum1/2
  Sum1/1 -> Gain2/1
  wl/1 -> Sum1/1, Unit Delay1/1
  wr/1 -> Sum/1, Unit Delay/1
  Sum/1 -> Gain1/1
  Unit Delay/1 -> Sum/2
  Gain1/1 -> Gain4/1
  Gain2/1 -> Gain5/1
  Add/1 -> Divide/1
  Constant/1 -> Divide/2
  Gain4/1 -> Add/1  "vr"
  Gain5/1 -> Add/2  "vl"
  Divide/1 -> w (deg/s)/1

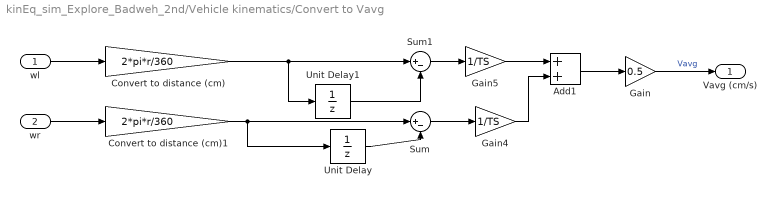
== system kinEq_sim_Explore_Badweh_2nd/Vehicle kinematics/Convert to Vavg ==
  wl : Inport
  wr : Inport  Port=2
  Add1 : Sum
  Convert to distance (cm) : Gain  Gain=2*pi*r/360
  Convert to distance (cm)1 : Gain  Gain=2*pi*r/360
  Gain : Gain  Gain=0.5
  Gain4 : Gain  Gain=1/TS
  Gain5 : Gain  Gain=1/TS
  Sum : Sum  Inputs=|+-
  Sum1 : Sum  Inputs=|+-
  Unit Delay : UnitDelay  SampleTime=-1  HasFrameUpgradeWarning=on
  Unit Delay1 : UnitDelay  SampleTime=-1  HasFrameUpgradeWarning=on
  Vavg (cm/s) : Outport  VectorParamsAs1DForOutWhenUnconnected=off
  wires:
  Gain/1 -> Vavg (cm/s)/1  "Vavg"
  Add1/1 -> Gain/1
  Unit Delay/1 -> Sum/2
  Sum/1 -> Gain4/1
  wr/1 -> Convert to distance (cm)1/1
  Gain4/1 -> Add1/2
  Gain5/1 -> Add1/1
  Sum1/1 -> Gain5/1
  Unit Delay1/1 -> Sum1/2
  wl/1 -> Convert to distance (cm)/1
  Convert to distance (cm)/1 -> Unit Delay1/1, Sum1/1
  Convert to distance (cm)1/1 -> Unit Delay/1, Sum/1

== system kinEq_sim_Explore_Badweh_2nd/Rover Simulation/ Encoder simulation/Encoder ==
  Lwheelspeed : Inport
  Rwheelspeed : Inport  Port=2
  Discrete-Time Integrator : DiscreteIntegrator  SampleTime=-1  ICPrevOutput=DiscIntNeverNeededParam  ICPrevScaledInput=DiscIntNeverNeededParam
  Discrete-Time Integrator1 : DiscreteIntegrator  SampleTime=-1  ICPrevOutput=DiscIntNeverNeededParam  ICPrevScaledInput=DiscIntNeverNeededParam
  LDegrees : Outport  VectorParamsAs1DForOutWhenUnconnected=off
  RDegrees : Outport  Port=2  VectorParamsAs1DForOutWhenUnconnected=off
  wires:
  Rwheelspeed/1 -> Discrete-Time Integrator/1
  Lwheelspeed/1 -> Discrete-Time Integrator1/1
  Discrete-Time Integrator/1 -> RDegrees/1
  Discrete-Time Integrator1/1 -> LDegrees/1

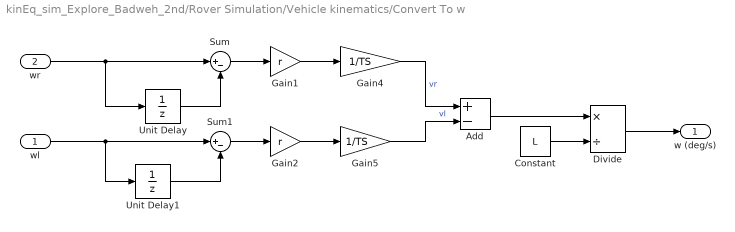
== system kinEq_sim_Explore_Badweh_2nd/Rover Simulation/Vehicle kinematics/Convert To w ==
  wl : Inport
  wr : Inport  Port=2
  Add : Sum  Inputs=+-
  Constant : Constant  Value=L
  Divide : Product  Inputs=*/
  Gain1 : Gain  Gain=r
  Gain2 : Gain  Gain=r
  Gain4 : Gain  Gain=1/TS
  Gain5 : Gain  Gain=1/TS
  Sum : Sum  Inputs=|+-
  Sum1 : Sum  Inputs=|+-
  Unit Delay : UnitDelay  SampleTime=-1  HasFrameUpgradeWarning=on
  Unit Delay1 : UnitDelay  SampleTime=-1  HasFrameUpgradeWarning=on
  w (deg/s) : Outport  VectorParamsAs1DForOutWhenUnconnected=off
  wires:
  Unit Delay1/1 -> Sum1/2
  Sum1/1 -> Gain2/1
  wl/1 -> Sum1/1, Unit Delay1/1
  wr/1 -> Sum/1, Unit Delay/1
  Sum/1 -> Gain1/1
  Unit Delay/1 -> Sum/2
  Gain1/1 -> Gain4/1
  Gain2/1 -> Gain5/1
  Add/1 -> Divide/1
  Constant/1 -> Divide/2
  Gain4/1 -> Add/1  "vr"
  Gain5/1 -> Add/2  "vl"
  Divide/1 -> w (deg/s)/1

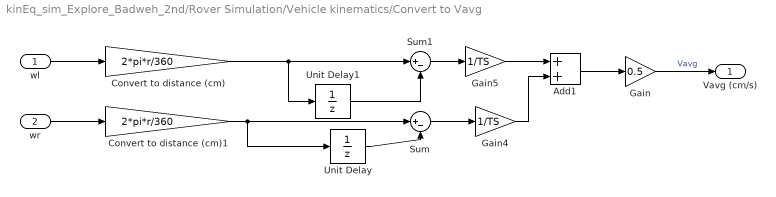
== system kinEq_sim_Explore_Badweh_2nd/Rover Simulation/Vehicle kinematics/Convert to Vavg ==
  wl : Inport
  wr : Inport  Port=2
  Add1 : Sum
  Convert to distance (cm) : Gain  Gain=2*pi*r/360
  Convert to distance (cm)1 : Gain  Gain=2*pi*r/360
  Gain : Gain  Gain=0.5
  Gain4 : Gain  Gain=1/TS
  Gain5 : Gain  Gain=1/TS
  Sum : Sum  Inputs=|+-
  Sum1 : Sum  Inputs=|+-
  Unit Delay : UnitDelay  SampleTime=-1  HasFrameUpgradeWarning=on
  Unit Delay1 : UnitDelay  SampleTime=-1  HasFrameUpgradeWarning=on
  Vavg (cm/s) : Outport  VectorParamsAs1DForOutWhenUnconnected=off
  wires:
  Gain/1 -> Vavg (cm/s)/1  "Vavg"
  Add1/1 -> Gain/1
  Unit Delay/1 -> Sum/2
  Sum/1 -> Gain4/1
  wr/1 -> Convert to distance (cm)1/1
  Gain4/1 -> Add1/2
  Gain5/1 -> Add1/1
  Sum1/1 -> Gain5/1
  Unit Delay1/1 -> Sum1/2
  wl/1 -> Convert to distance (cm)/1
  Convert to distance (cm)/1 -> Unit Delay1/1, Sum1/1
  Convert to distance (cm)1/1 -> Unit Delay/1, Sum/1

== matlab function kinEq_sim_Explore_Badweh_2nd/Rover Simulation/Robot path plotter/MATLAB Function  ==
  data: x input; y input; theta input; lineLength input; StartX parameter; StartY parameter; StartTheta parameter
function plotRobot(x,y,theta,lineLength, StartX, StartY, StartTheta)

% Create persistent variables for the figure windows
persistent h h1 h2;

if isempty(h)
    % Set up the initial figure window to display the initial position of
    % the rover
    h = figure('name','Map of the Robot');
    h1 = plot(StartX,StartY,'bo');
    hold on
    xlim([0 100])
    ylim([0 100])
    
    % Update the plot to show the heading of the rover
    xp = [StartX StartX+lineLength*cosd(StartTheta)];
    yp = [StartY StartY+lineLength*sind(StartTheta)];
    h2 = plot(xp,yp,'b');
    hold off
end

% Visualize the rover's path and heading
set(h1,'xdata',x,'ydata',y)
xp = [x x+lineLength*cosd(theta)];
yp = [y y+lineLength*sind(theta)];
set(h2,'xdata',xp,'ydata',yp)
drawnow('limitrate')

== matlab function kinEq_sim_Explore_Badweh_2nd/Rover Simulation/Vehicle kinematics/MATLAB Function  ==
  settings: updateMethod=DISCRETE  sampleTime=TS
  data: xprime output; yprime output; theta input; Vavg input
function [xprime, yprime] = vehiclesPath(theta, Vavg)
%#codegen

% Implement the equation for the real-world location of the rover
xprime = Vavg*cosd(theta);
yprime = Vavg*sind(theta);

== matlab function kinEq_sim_Explore_Badweh_2nd/MATLAB Function  ==
  data: x input; y input; theta input; lineLength input; StartX parameter; StartY parameter; StartTheta parameter
function plotRobot(x,y,theta,lineLength, StartX, StartY, StartTheta)

% Create persistent variables for the figure windows
persistent h h1 h2;

if isempty(h)
    % Set up the initial figure window to display the initial position of
    % the rover
    h = figure('name','Map of the Robot');
    h1 = plot(StartX,StartY,'bo');
    hold on
    xlim([0 100])
    ylim([0 100])
    
    % Update the plot to show the heading of the rover
    xp = [StartX StartX+lineLength*cosd(StartTheta)];
    yp = [StartY StartY+lineLength*sind(StartTheta)];
    h2 = plot(xp,yp,'b');
    hold off
end

% Visualize the rover's path and heading
set(h1,'xdata',x,'ydata',y)
xp = [x x+lineLength*cosd(theta)];
yp = [y y+lineLength*sind(theta)];
set(h2,'xdata',xp,'ydata',yp)
drawnow('limitrate')

== matlab function kinEq_sim_Explore_Badweh_2nd/MATLAB Function 1 ==
  settings: updateMethod=DISCRETE  sampleTime=TS
  data: xprime output; yprime output; theta input; Vavg input
function [xprime, yprime] = vehiclesPath(theta, Vavg)
%#codegen

% Implement the equation for the real-world location of the rover
xprime = Vavg*cosd(theta);
yprime = Vavg*sind(theta);

== matlab function kinEq_sim_Explore_Badweh_2nd/MATLAB Function 2 ==
  data: x input; y input; theta input; lineLength input; StartX parameter; StartY parameter; StartTheta parameter
function plotRobot(x,y,theta,lineLength, StartX, StartY, StartTheta)

% Create persistent variables for the figure windows
persistent h h1 h2;

if isempty(h)
    % Set up the initial figure window to display the initial position of
    % the rover
    h = figure('name','Map of the Robot');
    h1 = plot(StartX,StartY,'bo');
    hold on
    xlim([0 100])
    ylim([0 100])
    
    % Update the plot to show the heading of the rover
    xp = [StartX StartX+lineLength*cosd(StartTheta)];
    yp = [StartY StartY+lineLength*sind(StartTheta)];
    h2 = plot(xp,yp,'b');
    hold off
end

% Visualize the rover's path and heading
set(h1,'xdata',x,'ydata',y)
xp = [x x+lineLength*cosd(theta)];
yp = [y y+lineLength*sind(theta)];
set(h2,'xdata',xp,'ydata',yp)
drawnow('limitrate')

== matlab function kinEq_sim_Explore_Badweh_2nd/Vehicle kinematics/MATLAB Function  ==
  settings: updateMethod=DISCRETE  sampleTime=TS
  data: xprime output; yprime output; theta input; Vavg input
function [xprime, yprime] = vehiclesPath(theta, Vavg)
%#codegen

% Implement the equation for the real-world location of the rover
xprime = Vavg*cosd(theta);
yprime = Vavg*sind(theta);

== matlab function kinEq_sim_Explore_Badweh_2nd/MATLAB Function 3 ==
  settings: updateMethod=DISCRETE  sampleTime=TS
  data: xprime output; yprime output; theta input; Vavg input
function [xprime, yprime] = vehiclesPath(theta, Vavg)
%#codegen

% Implement the equation for the real-world location of the rover
xprime = Vavg*cosd(theta);
yprime = Vavg*sind(theta);

== matlab function kinEq_sim_Explore_Badweh_2nd/MATLAB Function 4 ==
  data: x input; y input; theta input; lineLength input; StartX parameter; StartY parameter; StartTheta parameter
function plotRobot(x,y,theta,lineLength, StartX, StartY, StartTheta)
% StartX = 50, StartY=20, StartTheta = 90 from matlab workspace
% Create persistent variables for the figure windows
persistent h h1 h2;

% initilize: run only once
if isempty(h)
    % Set up the initial figure window to display the initial position of
    % the rover
    disp('isempty')
    h = figure('name','Map of the Robot');
    h1 = plot(StartX,StartY,'bo');
    hold on
    xlim([0 100])
    ylim([0 100])

    % Update the plot to show the *heading* of the rover
    xp = [StartX StartX+lineLength*cosd(StartTheta)];
    yp = [StartY StartY+lineLength*sind(StartTheta)];
    h2 = plot(xp,yp,'r');
    hold off
end

% Visualize the rover's path and heading
set(h1,'xdata',x,'ydata',y) % position


 %heading
xp = [x x+lineLength*cosd(theta)];
yp = [y y+lineLength*sind(theta)];
set(h2,'xdata',xp,'ydata',yp)
drawnow('limitrate')
